simulink model "Coherent synchronous demodulator"  (R2022a)
settings: Solver=VariableStepAuto  StartTime=0.0  StopTime=50e-3  RelTol=1e-3
libraries: dspsrcs4 x5, dsparch4 x1
settings Model: Creator=Camille  LastModifiedBy=Camille

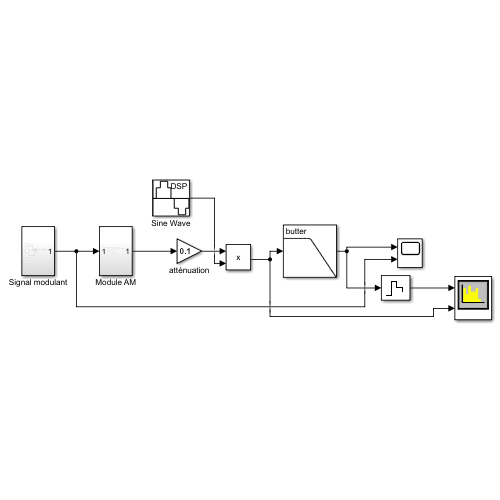
[thumbnail: Simulink's stored preview of the top-level diagram]
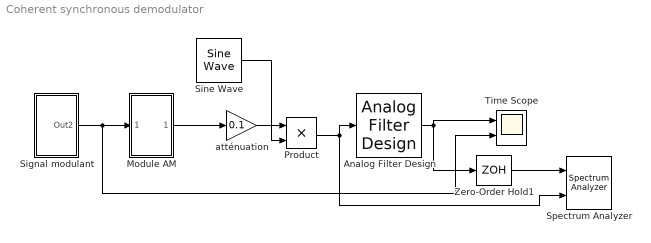
== system Coherent synchronous demodulator ==
  Analog Filter Design : dsparch4/Analog Filter Design  method=Butterworth  filttype=Lowpass  N=8  Wlo=63000  Whi=80  Rp=2  Rs=40
  Module AM : Subsystem
  Product : Product
  Signal modulant : Subsystem
  Sine Wave : dspsrcs4/Sine Wave  Amplitude=1  Frequency=20e3  Phase=pi/2  SampleMode=Discrete  OutComplex=Real  CompMethod=Trigonometric fcn  TableSize=Speed  SampleTime=1e-6  SamplesPerFrame=1  ResetState=Restart at time zero  OutputFrames=off  dataType=double  wordLen=16  udDataType=sfix(16)  fracBitsMode=Best precision  numFracBits=15  OutDataTypeStr=double  LastOutDataTypeStr=double
  Spectrum Analyzer : SpectrumAnalyzer  NumInputPorts=2
  Time Scope : Scope  NumInputPorts=2
  Zero-Order Hold1 : ZeroOrderHold  SampleTime=1e-6
  atténuation : Gain  Gain=0.1
  wires:
  Module AM/1(Out1) -> atténuation/1
  atténuation/1 -> Product/1
  Zero-Order Hold1/1 -> Spectrum Analyzer/1
  Product/1 -> Analog Filter Design/1, Spectrum Analyzer/2
  Signal modulant/1(Out2) -> Time Scope/2, Module AM/1(In1)
  Analog Filter Design/1 -> Time Scope/1, Zero-Order Hold1/1
  Sine Wave/1 -> Product/2

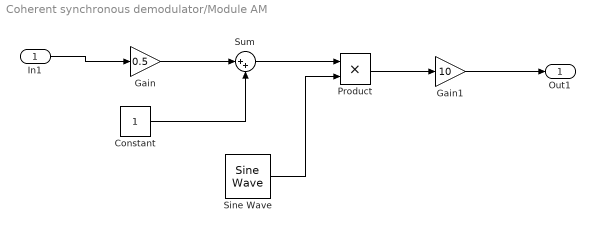
== system Coherent synchronous demodulator/Module AM ==
  In1 : Inport
  Constant : Constant
  Gain : Gain  Gain=0.5
  Gain1 : Gain  Gain=10
  Product : Product
  Sine Wave : dspsrcs4/Sine Wave  Amplitude=1  Frequency=20e3  Phase=pi/2  SampleMode=Discrete  OutComplex=Real  CompMethod=Trigonometric fcn  TableSize=Speed  SampleTime=0.1e-5  SamplesPerFrame=1  ResetState=Restart at time zero  OutputFrames=off  dataType=double  wordLen=16  udDataType=sfix(16)  fracBitsMode=Best precision  numFracBits=15  OutDataTypeStr=double  LastOutDataTypeStr=double
  Sum : Sum  Inputs=|++
  Out1 : Outport
  wires:
  Gain/1 -> Sum/1
  Gain1/1 -> Out1/1
  Constant/1 -> Sum/2
  Sine Wave/1 -> Product/2
  Sum/1 -> Product/1
  In1/1 -> Gain/1
  Product/1 -> Gain1/1

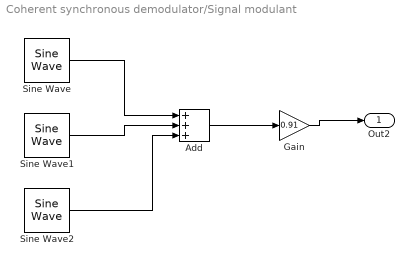
== system Coherent synchronous demodulator/Signal modulant ==
  Add : Sum  Inputs=+++
  Gain : Gain  Gain=0.91
  Sine Wave : dspsrcs4/Sine Wave  Amplitude=1  Frequency=0.5e3  Phase=0  SampleMode=Discrete  OutComplex=Real  CompMethod=Trigonometric fcn  TableSize=Speed  SampleTime=1e-6  SamplesPerFrame=1  ResetState=Restart at time zero  OutputFrames=off  dataType=double  wordLen=16  udDataType=sfix(16)  fracBitsMode=Best precision  numFracBits=15  OutDataTypeStr=double  LastOutDataTypeStr=double
  Sine Wave1 : dspsrcs4/Sine Wave  Amplitude=0.5  Frequency=1.5e3  Phase=0  SampleMode=Discrete  OutComplex=Real  CompMethod=Trigonometric fcn  TableSize=Speed  SampleTime=1e-6  SamplesPerFrame=1  ResetState=Restart at time zero  OutputFrames=off  dataType=double  wordLen=16  udDataType=sfix(16)  fracBitsMode=Best precision  numFracBits=15  OutDataTypeStr=double  LastOutDataTypeStr=double
  Sine Wave2 : dspsrcs4/Sine Wave  Amplitude=0.2  Frequency=2.5e3  Phase=0  SampleMode=Discrete  OutComplex=Real  CompMethod=Trigonometric fcn  TableSize=Speed  SampleTime=1e-6  SamplesPerFrame=1  ResetState=Restart at time zero  OutputFrames=off  dataType=double  wordLen=16  udDataType=sfix(16)  fracBitsMode=Best precision  numFracBits=15  OutDataTypeStr=double  LastOutDataTypeStr=double
  Out2 : Outport
  wires:
  Add/1 -> Gain/1
  Gain/1 -> Out2/1
  Sine Wave/1 -> Add/1
  Sine Wave1/1 -> Add/2
  Sine Wave2/1 -> Add/3
